simulink model "ofdm1"  (R2020b)
settings: Solver=FixedStepDiscrete  StartTime=0.0  StopTime=inf  RelTol=1e-3
PreLoadFcn:
  | N=64;
  | TsOFDM=4e-6;
InitFcn:
  | N=64;
  | TsOFDM=4e-6;
libraries: commrandsrc3 x1, commsink2 x1, dspxfrm3 x1, dspindex x1, commdigbbndpm3 x1
settings Model: Creator=ncavalier  LastModifiedBy=ncavalier
settings SolverCC: AutoInsertRateTranBlk=on
settings DataIOCC: LimitDataPoints=on  SaveOutput=off  SignalLogging=off  SaveTime=off
settings OptimizationCC: LifeSpan=inf  SimCompilerOptimization=on
settings DebuggingCC: AlgebraicLoopMsg=error  SingleTaskRateTransMsg=error  AllowSymbolicDim=off  SFUnexpectedBacktrackingDiag=warning  SFNoUnconditionalDefaultTransitionDiag=warning  SFExecutionAtInitializationDiag=none  ArithmeticOperatorsInVariantConditions=warning
settings SFSimCC: SimUseLocalCustomCode=off  CustomCodeUndefinedFunction=UseInterfaceOnly
settings RTWCC: RTWUseLocalCustomCode=off
settings CodeAppCC: StateflowObjectComments=on
settings GRTTargetCC: TargetLangStandard=C89/C90 (ANSI)
settings ConfigComp: CovMetricSettings=dw  CovSaveCumulativeToWorkspaceVar=on  CovSaveSingleToWorkspaceVar=on  CovExternalEMLEnable=off  CovSFcnEnable=off

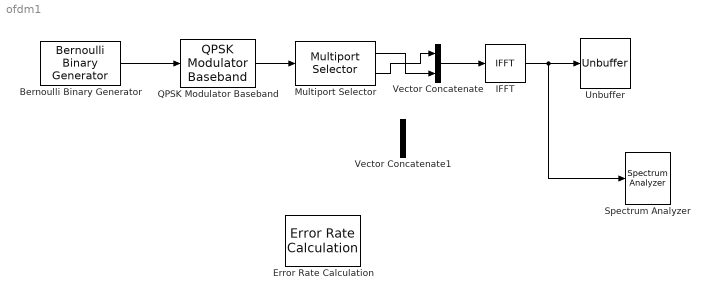
== system ofdm1 ==
  Bernoulli Binary Generator : commrandsrc3/Bernoulli Binary Generator  ProbabilityOfZero=0.5  SeedSource=Parameter  Seed=randi(1000)  SampleTime=TsOFDM/(2*N)  SamplesPerFrame=2*N  OutputDataType=double  SimulateUsing=Code generation
  Error Rate Calculation : commsink2/Error Rate Calculation  N=0  st_delay=0  cp_mode=Entire frame  subframe=[]  PMode=Workspace  WsName=ErrorVec  RsMode2=off  stop=off  numErr=100  maxBits=1e6
      settings: SourceProductName=Communications Toolbox
  IFFT : dspxfrm3/IFFT  FFTImplementation=Auto  CompMethod=Table lookup  TableOpt=NEW  TableOptActive=Speed  BitRevOrder=off  cs_in=off  Normalize=on  InheritFFTLength=on  FFTLength=64  WrapInput=on  mode=Complex  outSamplingMode=Sample based  roundingMode=Floor  overflowMode=off  firstCoeffDataTypeStr=Inherit: Same word length as input  firstCoeffLastDataTypeStr=Inherit: Same word length as input  outputMin=[]  outputMax=[]
  Multiport Selector : dspindex/Multiport Selector  rowsOrCols=Rows  idxCellArray={ 1 : N/2, (N/2) + 1 : N}  idxErrMode=Clip Index
  QPSK Modulator Baseband : commdigbbndpm3/QPSK Modulator Baseband  InType=Bit  Enc=Gray  Ph=pi/4  outDtype=double  outWordLen=16  outUDDataType=sfix(16)  outFracLenMode=Best precision  outFracLen=15  outDataTypeStr=double  outLastDataTypeStr=double
      settings: SourceProductName=Communications Toolbox
  Spectrum Analyzer : SpectrumAnalyzer
  Unbuffer : Unbuffer
  Vector Concatenate : Concatenate
  Vector Concatenate1 : Concatenate
  wires:
  Bernoulli Binary Generator/1 -> QPSK Modulator Baseband/1
  QPSK Modulator Baseband/1 -> Multiport Selector/1
  Multiport Selector/1 -> Vector Concatenate/2
  Multiport Selector/2 -> Vector Concatenate/1
  Vector Concatenate/1 -> IFFT/1
  IFFT/1 -> Spectrum Analyzer/1, Unbuffer/1
